simulink model "sim_att_dist_obs_tie_2020"  (R2020a)
settings: Solver=ode4  StartTime=0.0  StopTime=30.0  FixedStep=0.01  RelTol=1e-3
values from neighbouring files (symbols this model uses):
  beta_Phi_1 = pp0 * cal_frac_squ( 3, p_p0_plus_1, q_p0_plus_1 )                          * cal_frac_squ( eps_s_bar / pi, p_p0_min_2, q_p0_min_2 )                          / ( 2 * ( 2 * pp0 - 1 ) * tanh( gamma0 * ( eps_s_bar / pi ) / 2 ) )                          - ( cal_frac_squ( 3, p_p0_plus_1, q_p0_plus_1 ) * gamma0 / ( 4 * ( 2 * pp0 -1 ) ) )                          * cal_frac_squ( eps_s_bar / pi, p_p0_min_ ...(+136 chars)    [init_att_dist_obs_tie_2020.m]
  beta_Phi_2 = ( 1 - pp0 ) * cal_frac_squ( 3, p_p0_plus_1, q_p0_plus_1 )                          / ( 2 * ( 1 - 2 * pp0 ) * cal_frac_squ( eps_s_bar / pi, p_p0_0, q_p0_0 ) * tanh( gamma0 * ( eps_s_bar / pi ) / 2 ) )                          - ( cal_frac_squ( 3, p_p0_plus_1, q_p0_plus_1 ) * gamma0 / ( 4 * ( 1 - 2 * pp0 ) ) )                          * cal_frac_squ( eps_s_bar / pi, p_1_min_p0, q_1_min_p0 )          ...(+112 chars)    [init_att_dist_obs_tie_2020.m]
  c1_diff_ui = diag([25; 30; 20])    [init_att_dist_obs_tie_2020.m]
  c2_diff_ui = diag([50; 50; 10])    [init_att_dist_obs_tie_2020.m]
  c3_diff_ui = diag([15; 15; 10])    [init_att_dist_obs_tie_2020.m]
  c_w_1 = diag( [20; 15; 15] )    [init_att_dist_obs_tie_2020.m]
  c_w_2 = diag( [20; 15; 15] )    [init_att_dist_obs_tie_2020.m]
  c_w_3 = diag( [2; 2; 2] )    [init_att_dist_obs_tie_2020.m]
  cS0 = diag( [4.5; 4.5; 4.5] )    [init_att_dist_obs_tie_2020.m]
  dw_aa_t = 0.2 * ones(3, 5) + ( 1.0 - 0.2 ) * rand(3, 5)    [init_att_dist_obs_tie_2020.m]
  dw_ff_t = [ 0.4 * ones(1, 5) + ( 1.0 - 0.4 ) * rand(1, 5);                      0.4 * ones(1, 5) + ( 1.0 - 0.4 ) * rand(1, 5);                      0.2 * ones(1, 5) + ( 0.6 - 0.2 ) * rand(1, 5) ]    [init_att_dist_obs_tie_2020.m]
  dw_phi_t = ( - pi / 2 ) * ones(3, 5) + ( pi / 2 - ( - pi / 2 ) ) * rand(3, 5)    [init_att_dist_obs_tie_2020.m]
  dwci_init = zeros(3,5)    [init_att_dist_obs_tie_2020.m]
  eps_s_bar_div_pi = eps_s_bar / pi    (= 0.03)    [init_att_dist_obs_tie_2020.m]
  epw = [1; 1; 1]    [init_att_dist_obs_tie_2020.m]
  gamma0 = 20    [init_att_dist_obs_tie_2020.m]
  Ji = zeros(3,3,NF)    [init_att_dist_obs_tie_2020.m]
  k_J_0 = diag( [1; 1; 1] )    [init_att_dist_obs_tie_2020.m]
  kaiw = [10; 10; 10]    [init_att_dist_obs_tie_2020.m]
  l1w = [50; 50; 50]    [init_att_dist_obs_tie_2020.m]
  l2w = [60; 60; 60]    [init_att_dist_obs_tie_2020.m]
  Lamd_diff_ui = 0.8    [init_att_dist_obs_tie_2020.m]
  mu_c_theta = 100    [init_att_dist_obs_tie_2020.m]
  pos0 = zeros(3, 1)    [init_att_dist_obs_tie_2020.m]
  pp0 = 8 / 11    (= 0.727272727273)    [init_att_dist_obs_tie_2020.m]
  PZ0 = P0(3)    [init_att_dist_obs_tie_2020.m]
  PZ1 = 10    [init_att_dist_obs_tie_2020.m]
  Qci_init = repmat([1;0;0;0],1,NF)    [init_att_dist_obs_tie_2020.m]
  R0 = 4    [init_att_dist_obs_tie_2020.m]
  R1 = 8    [init_att_dist_obs_tie_2020.m]
  Rci_init = zeros(3,3,NF)    [init_att_dist_obs_tie_2020.m]
  Ri_init = zeros(3,3,NF)    [init_att_dist_obs_tie_2020.m]
  Rx2 = 10    [init_att_dist_obs_tie_2020.m]
  Ry2 = 6    [init_att_dist_obs_tie_2020.m]
  Rz2 = 4    [init_att_dist_obs_tie_2020.m]
  T0 = 0    [init_att_dist_obs_tie_2020.m]
  T1 = tseq1    (= 10)    [init_att_dist_obs_tie_2020.m]
  T2 = tseq1 + tseq12 + tseq2    (= 30)    [init_att_dist_obs_tie_2020.m]
  thr_p_plus_1 = cal_frac_squ( 3, p_p0_plus_1, q_p0_plus_1 )    [init_att_dist_obs_tie_2020.m]
  ui_init = zeros(3,NF)    [init_att_dist_obs_tie_2020.m]
  vel0 = zeros(3, 1)    [init_att_dist_obs_tie_2020.m]
  wci_init = zeros(3,5)    [init_att_dist_obs_tie_2020.m]
  zeta_diff_ui = 0.05    [init_att_dist_obs_tie_2020.m]
undefined symbols (not defined in the file or in its folder): cal_frac_squ, p_2_p0, p_beta_w_1, p_beta_w_2, p_p0_min_1, p_p0_plus_1, q_2_p0, q_beta_w_1, q_beta_w_2, q_p0_min_1, q_p0_plus_1, Qei_init, Qi_init, Rei_init, V_Phi_Rei_init, wei_init, wi_init
(part 3 of 4)

== matlab function sim_att_dist_obs_tie_2020/combine V_Phi_Rei_squ_2p ==
  data: V_Phi_Rei_squ_2p_node_1 input; V_Phi_Rei_squ_2p_node_2 input; V_Phi_Rei_squ_2p_node_3 input; V_Phi_Rei_squ_2p_node_4 input; V_Phi_Rei_squ_2p_node_5 input; V_Phi_Rei_squ_2p_vec output
function V_Phi_Rei_squ_2p_vec  = fcn(V_Phi_Rei_squ_2p_node_1, V_Phi_Rei_squ_2p_node_2, V_Phi_Rei_squ_2p_node_3, ...
                                                                        V_Phi_Rei_squ_2p_node_4, V_Phi_Rei_squ_2p_node_5)
%%%% 合并姿态误差指数坐标
V_Phi_Rei_squ_2p_vec = zeros(3,5);
V_Phi_Rei_squ_2p_vec(:,1) = V_Phi_Rei_squ_2p_node_1(:);
V_Phi_Rei_squ_2p_vec(:,2) = V_Phi_Rei_squ_2p_node_2(:);
V_Phi_Rei_squ_2p_vec(:,3) = V_Phi_Rei_squ_2p_node_3(:);
V_Phi_Rei_squ_2p_vec(:,4) = V_Phi_Rei_squ_2p_node_4(:);
V_Phi_Rei_squ_2p_vec(:,5) = V_Phi_Rei_squ_2p_node_5(:);

== matlab function sim_att_dist_obs_tie_2020/combine V_Phi_Rei_squ_p_min_1 ==
  data: V_Phi_Rei_squ_p_min_1_node_1 input; V_Phi_Rei_squ_p_min_1_node_2 input; V_Phi_Rei_squ_p_min_1_node_3 input; V_Phi_Rei_squ_p_min_1_node_4 input; V_Phi_Rei_squ_p_min_1_node_5 input; V_Phi_Rei_squ_p_min_1_vec output
function V_Phi_Rei_squ_p_min_1_vec  = fcn(V_Phi_Rei_squ_p_min_1_node_1, V_Phi_Rei_squ_p_min_1_node_2, V_Phi_Rei_squ_p_min_1_node_3, ...
                                                                                V_Phi_Rei_squ_p_min_1_node_4, V_Phi_Rei_squ_p_min_1_node_5)
%%%% 合并姿态误差导数
V_Phi_Rei_squ_p_min_1_vec = zeros(3,5);
V_Phi_Rei_squ_p_min_1_vec(:,1) = V_Phi_Rei_squ_p_min_1_node_1(:);
V_Phi_Rei_squ_p_min_1_vec(:,2) = V_Phi_Rei_squ_p_min_1_node_2(:);
V_Phi_Rei_squ_p_min_1_vec(:,3) = V_Phi_Rei_squ_p_min_1_node_3(:);
V_Phi_Rei_squ_p_min_1_vec(:,4) = V_Phi_Rei_squ_p_min_1_node_4(:);
V_Phi_Rei_squ_p_min_1_vec(:,5) = V_Phi_Rei_squ_p_min_1_node_5(:);

== matlab function sim_att_dist_obs_tie_2020/cal neso x1_hat agent 3 ==
  data: l1w input; epw input; Ji input; x1_hat_vec input; dw_hat_vec input; wi_vec input; d_x1_hat_3 output; taui_vec input
function d_x1_hat_3 = fcn(l1w, epw, Ji, x1_hat_vec, dw_hat_vec, wi_vec, taui_vec)
%%%% 计算扰动观测中间变量
iiuav = 3;
d_x1_hat_3 = dw_hat_vec(:,iiuav) + (l1w ./ epw) .* (Ji(:,:,iiuav) * wi_vec(:,iiuav) - x1_hat_vec(:,iiuav)) ...
                        + ( -cal_askew_mat(wi_vec(:,iiuav)) * Ji(:,:,iiuav) * wi_vec(:,iiuav) + taui_vec(:,iiuav) );

== matlab function sim_att_dist_obs_tie_2020/combine V_Phi_Rei_squ_p_plus_1 ==
  data: V_Phi_Rei_squ_p_plus_1_node_1 input; V_Phi_Rei_squ_p_plus_1_node_2 input; V_Phi_Rei_squ_p_plus_1_node_3 input; V_Phi_Rei_squ_p_plus_1_node_4 input; V_Phi_Rei_squ_p_plus_1_node_5 input; V_Phi_Rei_squ_p_plus_1_vec output
function V_Phi_Rei_squ_p_plus_1_vec  = fcn(V_Phi_Rei_squ_p_plus_1_node_1, V_Phi_Rei_squ_p_plus_1_node_2, V_Phi_Rei_squ_p_plus_1_node_3, ...
                                                                                V_Phi_Rei_squ_p_plus_1_node_4, V_Phi_Rei_squ_p_plus_1_node_5)
%%%% 合并姿态误差指数坐标
V_Phi_Rei_squ_p_plus_1_vec = zeros(3,5);
V_Phi_Rei_squ_p_plus_1_vec(:,1) = V_Phi_Rei_squ_p_plus_1_node_1(:);
V_Phi_Rei_squ_p_plus_1_vec(:,2) = V_Phi_Rei_squ_p_plus_1_node_2(:);
V_Phi_Rei_squ_p_plus_1_vec(:,3) = V_Phi_Rei_squ_p_plus_1_node_3(:);
V_Phi_Rei_squ_p_plus_1_vec(:,4) = V_Phi_Rei_squ_p_plus_1_node_4(:);
V_Phi_Rei_squ_p_plus_1_vec(:,5) = V_Phi_Rei_squ_p_plus_1_node_5(:);

== matlab function sim_att_dist_obs_tie_2020/combine duihat d2uihat ==
  data: d_ui_hat_node_1 input; duihat_vec output; d2uihat_vec output; d_ui_hat_node_2 input; d_ui_hat_node_3 input; d_ui_hat_node_4 input; d_ui_hat_node_5 input; d2_ui_hat_node_1 input; d2_ui_hat_node_2 input; d2_ui_hat_node_3 input; d2_ui_hat_node_4 input; d2_ui_hat_node_5 input
function [duihat_vec, d2uihat_vec] = fcn(d_ui_hat_node_1, d_ui_hat_node_2, d_ui_hat_node_3, d_ui_hat_node_4, d_ui_hat_node_5, ...
                                                                            d2_ui_hat_node_1, d2_ui_hat_node_2, d2_ui_hat_node_3, d2_ui_hat_node_4, d2_ui_hat_node_5)

duihat_vec = [d_ui_hat_node_1(:), d_ui_hat_node_2(:), d_ui_hat_node_3(:), d_ui_hat_node_4(:), d_ui_hat_node_5(:)];
d2uihat_vec = [d2_ui_hat_node_1(:), d2_ui_hat_node_2(:), d2_ui_hat_node_3(:), d2_ui_hat_node_4(:), d2_ui_hat_node_5(:)];

== matlab function sim_att_dist_obs_tie_2020/combine dwi ==
  data: wi_1 input; wi_vec output; wi_2 input; wi_3 input; wi_4 input; wi_5 input
function wi_vec = fcn(wi_1, wi_2, wi_3, wi_4, wi_5)
%%%% 合并姿态角速率
wi_vec = [wi_1(:), wi_2(:), wi_3(:), wi_4(:), wi_5(:)];

== matlab function sim_att_dist_obs_tie_2020/combine tau ==
  data: tau_1 input; taui_vec output; tau_2 input; tau_3 input; tau_4 input; tau_5 input
function taui_vec = fcn(tau_1, tau_2, tau_3, tau_4, tau_5)
%%%% 合并辅助姿态角速率
taui_vec = [tau_1(:), tau_2(:), tau_3(:), tau_4(:), tau_5(:)];

== matlab function sim_att_dist_obs_tie_2020/combine tau1 ==
  data: dw_1 input; dw_vec output; dw_2 input; dw_3 input; dw_4 input; dw_5 input
function dw_vec = fcn(dw_1, dw_2, dw_3, dw_4, dw_5)
%%%% 合并辅助姿态角速率
dw_vec = [dw_1(:), dw_2(:), dw_3(:), dw_4(:), dw_5(:)];

== matlab function sim_att_dist_obs_tie_2020/combine theta_Si_beta_w_1 ==
  data: theta_Si_beta_w_1_node_1 input; theta_Si_beta_w_1_node_2 input; theta_Si_beta_w_1_node_3 input; theta_Si_beta_w_1_node_4 input; theta_Si_beta_w_1_node_5 input; theta_Si_beta_w_1_vec output
function theta_Si_beta_w_1_vec  = fcn(theta_Si_beta_w_1_node_1, theta_Si_beta_w_1_node_2, theta_Si_beta_w_1_node_3, ...
                                                                        theta_Si_beta_w_1_node_4, theta_Si_beta_w_1_node_5)
%%%% 合并误差非线性项
theta_Si_beta_w_1_vec = zeros(3,5);
theta_Si_beta_w_1_vec(:,1) = theta_Si_beta_w_1_node_1(:);
theta_Si_beta_w_1_vec(:,2) = theta_Si_beta_w_1_node_2(:);
theta_Si_beta_w_1_vec(:,3) = theta_Si_beta_w_1_node_3(:);
theta_Si_beta_w_1_vec(:,4) = theta_Si_beta_w_1_node_4(:);
theta_Si_beta_w_1_vec(:,5) = theta_Si_beta_w_1_node_5(:);

== matlab function sim_att_dist_obs_tie_2020/combine theta_Si_beta_w_2 ==
  data: theta_Si_beta_w_2_node_1 input; theta_Si_beta_w_2_node_2 input; theta_Si_beta_w_2_node_3 input; theta_Si_beta_w_2_node_4 input; theta_Si_beta_w_2_node_5 input; theta_Si_beta_w_2_vec output
function theta_Si_beta_w_2_vec  = fcn(theta_Si_beta_w_2_node_1, theta_Si_beta_w_2_node_2, theta_Si_beta_w_2_node_3, ...
                                                                        theta_Si_beta_w_2_node_4, theta_Si_beta_w_2_node_5)
%%%% 合并误差非线性项
theta_Si_beta_w_2_vec = zeros(3,5);
theta_Si_beta_w_2_vec(:,1) = theta_Si_beta_w_2_node_1(:);
theta_Si_beta_w_2_vec(:,2) = theta_Si_beta_w_2_node_2(:);
theta_Si_beta_w_2_vec(:,3) = theta_Si_beta_w_2_node_3(:);
theta_Si_beta_w_2_vec(:,4) = theta_Si_beta_w_2_node_4(:);
theta_Si_beta_w_2_vec(:,5) = theta_Si_beta_w_2_node_5(:);

== matlab function sim_att_dist_obs_tie_2020/combine wci dwci ==
  data: wci_node_1 input; wci_vec output; wci_node_2 input; wci_node_3 input; wci_node_4 input; wci_node_5 input; dwci_vec output; dwci_node_1 input; dwci_node_2 input; dwci_node_3 input; dwci_node_4 input; dwci_node_5 input
function [wci_vec, dwci_vec] = fcn(wci_node_1, wci_node_2, wci_node_3, wci_node_4, wci_node_5, ...
                                                                dwci_node_1, dwci_node_2, dwci_node_3, dwci_node_4, dwci_node_5)
%%%% 合并姿态角速率指令及其导数
wci_vec = [wci_node_1(:), wci_node_2(:), wci_node_3(:), wci_node_4(:), wci_node_5(:)];
dwci_vec = [dwci_node_1(:), dwci_node_2(:), dwci_node_3(:), dwci_node_4(:), dwci_node_5(:)];

== matlab function sim_att_dist_obs_tie_2020/combine wei Qei Rei ==
  data: wei_1 input; wei_vec output; wei_2 input; wei_3 input; wei_4 input; wei_5 input; Qei_1 input; Qei_2 input; Qei_3 input; Qei_4 input; Qei_5 input; Rei_1 input; Rei_2 input; Rei_3 input; Rei_4 input; Rei_5 input; Qei_vec output; Rei_vec output
function [wei_vec, Qei_vec, Rei_vec] = fcn(wei_1, wei_2, wei_3, wei_4, wei_5, ...
                                                                            Qei_1, Qei_2, Qei_3, Qei_4, Qei_5, ...
                                                                            Rei_1, Rei_2, Rei_3, Rei_4, Rei_5)
%%%% 合并姿态角速率误差/四元数误差/姿态旋转矩阵误差
wei_vec = zeros(3,5);
wei_vec(:,1) = wei_1(:);
wei_vec(:,2) = wei_2(:);
wei_vec(:,3) = wei_3(:);
wei_vec(:,4) = wei_4(:);
wei_vec(:,5) = wei_5(:);

Qei_vec = zeros(4,5);
Qei_vec(:,1) = Qei_1(:);
Qei_vec(:,2) = Qei_2(:);
Qei_vec(:,3) = Qei_3(:);
Qei_vec(:,4) = Qei_4(:);
Qei_vec(:,5) = Qei_5(:);

Rei_vec = zeros(3,3,5);
Rei_vec(:,:,1) = Rei_1;
Rei_vec(:,:,2) = Rei_2;
Rei_vec(:,:,3) = Rei_3;
Rei_vec(:,:,4) = Rei_4;
Rei_vec(:,:,5) = Rei_5;

== matlab function sim_att_dist_obs_tie_2020/cal neso x1_hat agent 4 ==
  data: l1w input; epw input; Ji input; x1_hat_vec input; dw_hat_vec input; wi_vec input; d_x1_hat_4 output; taui_vec input
function d_x1_hat_4 = fcn(l1w, epw, Ji, x1_hat_vec, dw_hat_vec, wi_vec, taui_vec)
%%%% 计算扰动观测中间变量
iiuav = 4;
d_x1_hat_4 = dw_hat_vec(:,iiuav) + (l1w ./ epw) .* (Ji(:,:,iiuav) * wi_vec(:,iiuav) - x1_hat_vec(:,iiuav)) ...
                        + ( -cal_askew_mat(wi_vec(:,iiuav)) * Ji(:,:,iiuav) * wi_vec(:,iiuav) + taui_vec(:,iiuav) );

== matlab function sim_att_dist_obs_tie_2020/generate angular rate disturbance agent 1 ==
  data: dw_1 output; dw_aa_t input; dw_ff_t input; dw_phi_t input; t input
function dw_1 = fcn(dw_aa_t, dw_ff_t, dw_phi_t, t)
%%%% 姿态动力学方程中的扰动项设置
epsil_t = zeros(3, 1);

for kk = 1:5
    epsil_t = epsil_t + dw_aa_t(:, kk) .* sin( 2 * pi * dw_ff_t(:, kk) * t + dw_phi_t(:, kk) );
end

dw_1 = [ epsil_t(1) + 1.6 * sin( 0.4 * t ) + 2.0 * cos( 0.5 * t ) + 1.4 * sin( 0.7 * t ) ...
                + 4 * exp( -0.1 * t ) * sin( 0.8 * t ) + 3 / ( 1 + exp( -0.2 * ( t - 15 ) ) ); ...
                epsil_t(2) + 1.2 * sin( 0.2 * t ) + 3 * cos( 0.4 * t ) + 0.8 * sin( 0.6 * t ) ...
                + 2 * exp( -0.15 * t ) * cos( 1.2 * t ) + 3 / ( 1 + exp( -0.3 * ( t - 25 ) ) ); ...
                epsil_t(3) + 1.8 * sin( 0.2 * t ) + 1.6 * sin( 0.3 * t ) + 1.6 * cos( 0.4 * t ) ...
                + 4 * exp( -0.05 * t ) * sin( 0.5 * t + pi / 4 ) + 3 / ( 1 + exp( -0.5 * ( t - 20 ) ) ) ];

== matlab function sim_att_dist_obs_tie_2020/generate angular rate disturbance agent 2 ==
  data: dw_2 output; dw_aa_t input; dw_ff_t input; dw_phi_t input; t input
function dw_2 = fcn(dw_aa_t, dw_ff_t, dw_phi_t, t)
%%%% 姿态动力学方程中的扰动项设置
epsil_t = zeros(3, 1);

for kk = 1:5
    epsil_t = epsil_t + dw_aa_t(:, kk) .* sin( 2 * pi * dw_ff_t(:, kk) * t + dw_phi_t(:, kk) );
end

dw_2 = [ epsil_t(1) + 1.6 * sin( 0.2 * t ) + 2.0 * cos( 0.3 * t ) + 1.4 * sin( 0.5 * t ) ...
                + 4 * exp( -0.1 * t ) * sin( 0.5 * t ) + 3 / ( 1 + exp( -0.2 * ( t - 15 ) ) ); ...
                epsil_t(2) + 1.2 * sin( 0.1 * t ) + 3 * cos( 0.2 * t ) + 0.8 * sin( 0.4 * t ) ...
                + 2 * exp( -0.15 * t ) * cos( 0.6 * t ) + 3 / ( 1 + exp( -0.3 * ( t - 25 ) ) ); ...
                epsil_t(3) + 1.8 * sin( 0.1 * t ) + 1.6 * sin( 0.2 * t ) + 1.6 * cos( 0.3 * t ) ...
                + 4 * exp( -0.05 * t ) * sin( 0.4 * t + pi / 4 ) + 3 / ( 1 + exp( -0.5 * ( t - 20 ) ) ) ];

== matlab function sim_att_dist_obs_tie_2020/generate angular rate disturbance agent 3 ==
  data: dw_3 output; dw_aa_t input; dw_ff_t input; dw_phi_t input; t input
function dw_3 = fcn(dw_aa_t, dw_ff_t, dw_phi_t, t)
%%%% 姿态动力学方程中的扰动项设置
epsil_t = zeros(3, 1);

for kk = 1:5
    epsil_t = epsil_t + dw_aa_t(:, kk) .* sin( 2 * pi * dw_ff_t(:, kk) * t + dw_phi_t(:, kk) );
end

dw_3 = [ epsil_t(1) + 1.6 * sin( 0.2 * t ) + 2.0 * cos( 0.3 * t ) + 1.4 * sin( 0.5 * t ) ...
                + 4 * exp( -0.1 * t ) * sin( 0.5 * t ) + 3 / ( 1 + exp( -0.2 * ( t - 15 ) ) ); ...
                epsil_t(2) + 1.2 * sin( 0.1 * t ) + 3 * cos( 0.2 * t ) + 0.8 * sin( 0.4 * t ) ...
                + 2 * exp( -0.15 * t ) * cos( 0.6 * t ) + 3 / ( 1 + exp( -0.3 * ( t - 25 ) ) ); ...
                epsil_t(3) + 1.8 * sin( 0.1 * t ) + 1.6 * sin( 0.2 * t ) + 1.6 * cos( 0.3 * t ) ...
                + 4 * exp( -0.05 * t ) * sin( 0.4 * t + pi / 4 ) + 3 / ( 1 + exp( -0.5 * ( t - 20 ) ) ) ];

== matlab function sim_att_dist_obs_tie_2020/generate angular rate disturbance agent 4 ==
  data: dw_4 output; dw_aa_t input; dw_ff_t input; dw_phi_t input; t input
function dw_4 = fcn(dw_aa_t, dw_ff_t, dw_phi_t, t)
%%%% 姿态动力学方程中的扰动项设置
epsil_t = zeros(3, 1);

for kk = 1:5
    epsil_t = epsil_t + dw_aa_t(:, kk) .* sin( 2 * pi * dw_ff_t(:, kk) * t + dw_phi_t(:, kk) );
end

dw_4 = [ epsil_t(1) + 1.6 * sin( 0.2 * t ) + 2.0 * cos( 0.3 * t ) + 1.4 * sin( 0.5 * t ) ...
                + 4 * exp( -0.1 * t ) * sin( 0.5 * t ) + 3 / ( 1 + exp( -0.2 * ( t - 15 ) ) ); ...
                epsil_t(2) + 1.2 * sin( 0.1 * t ) + 3 * cos( 0.2 * t ) + 0.8 * sin( 0.4 * t ) ...
                + 2 * exp( -0.15 * t ) * cos( 0.6 * t ) + 3 / ( 1 + exp( -0.3 * ( t - 25 ) ) ); ...
                epsil_t(3) + 1.8 * sin( 0.1 * t ) + 1.6 * sin( 0.2 * t ) + 1.6 * cos( 0.3 * t ) ...
                + 4 * exp( -0.05 * t ) * sin( 0.4 * t + pi / 4 ) + 3 / ( 1 + exp( -0.5 * ( t - 20 ) ) ) ];

== matlab function sim_att_dist_obs_tie_2020/generate angular rate disturbance agent 5 ==
  data: dw_5 output; dw_aa_t input; dw_ff_t input; dw_phi_t input; t input
function dw_5 = fcn(dw_aa_t, dw_ff_t, dw_phi_t, t)
%%%% 姿态动力学方程中的扰动项设置
epsil_t = zeros(3, 1);

for kk = 1:5
    epsil_t = epsil_t + dw_aa_t(:, kk) .* sin( 2 * pi * dw_ff_t(:, kk) * t + dw_phi_t(:, kk) );
end

dw_5 = [ epsil_t(1) + 1.6 * sin( 0.2 * t ) + 2.0 * cos( 0.3 * t ) + 1.4 * sin( 0.5 * t ) ...
                + 4 * exp( -0.1 * t ) * sin( 0.5 * t ) + 3 / ( 1 + exp( -0.2 * ( t - 15 ) ) ); ...
                epsil_t(2) + 1.2 * sin( 0.1 * t ) + 3 * cos( 0.2 * t ) + 0.8 * sin( 0.4 * t ) ...
                + 2 * exp( -0.15 * t ) * cos( 0.6 * t ) + 3 / ( 1 + exp( -0.3 * ( t - 25 ) ) ); ...
                epsil_t(3) + 1.8 * sin( 0.1 * t ) + 1.6 * sin( 0.2 * t ) + 1.6 * cos( 0.3 * t ) ...
                + 4 * exp( -0.05 * t ) * sin( 0.4 * t + pi / 4 ) + 3 / ( 1 + exp( -0.5 * ( t - 20 ) ) ) ];

== matlab function sim_att_dist_obs_tie_2020/trans to column100 ==
  data: x input; y output
function y = fcn(x)
y = x(:);

== matlab function sim_att_dist_obs_tie_2020/trans to column101 ==
  data: x input; y output
function y = fcn(x)
y = x(:);

== matlab function sim_att_dist_obs_tie_2020/trans to column102 ==
  data: x input; y output
function y = fcn(x)
y = x(:);

== matlab function sim_att_dist_obs_tie_2020/trans to column103 ==
  data: x input; y output
function y = fcn(x)
y = x(:);

== matlab function sim_att_dist_obs_tie_2020/trans to column104 ==
  data: x input; y output
function y = fcn(x)
y = x(:);

== matlab function sim_att_dist_obs_tie_2020/trans to column105 ==
  data: x input; y output
function y = fcn(x)
y = x(:);

== matlab function sim_att_dist_obs_tie_2020/trans to column106 ==
  data: x input; y output
function y = fcn(x)
y = x(:);

== matlab function sim_att_dist_obs_tie_2020/trans to column116 ==
  data: x input; y output
function y = fcn(x)
y = x(:);

== matlab function sim_att_dist_obs_tie_2020/trans to column118 ==
  data: x input; y output
function y = fcn(x)
y = x(:);

== matlab function sim_att_dist_obs_tie_2020/trans to column119 ==
  data: x input; y output
function y = fcn(x)
y = x(:);

== matlab function sim_att_dist_obs_tie_2020/trans to column120 ==
  data: x input; y output
function y = fcn(x)
y = x(:);

== matlab function sim_att_dist_obs_tie_2020/trans to column121 ==
  data: x input; y output
function y = fcn(x)
y = x(:);

== matlab function sim_att_dist_obs_tie_2020/cal neso x1_hat agent 5 ==
  data: l1w input; epw input; Ji input; x1_hat_vec input; dw_hat_vec input; wi_vec input; d_x1_hat_5 output; taui_vec input
function d_x1_hat_5 = fcn(l1w, epw, Ji, x1_hat_vec, dw_hat_vec, wi_vec, taui_vec)
%%%% 计算扰动观测中间变量
iiuav = 5;
d_x1_hat_5 = dw_hat_vec(:,iiuav) + (l1w ./ epw) .* (Ji(:,:,iiuav) * wi_vec(:,iiuav) - x1_hat_vec(:,iiuav)) ...
                        + ( -cal_askew_mat(wi_vec(:,iiuav)) * Ji(:,:,iiuav) * wi_vec(:,iiuav) + taui_vec(:,iiuav) );

== matlab function sim_att_dist_obs_tie_2020/trans to column122 ==
  data: x input; y output
function y = fcn(x)
y = x(:);

== matlab function sim_att_dist_obs_tie_2020/trans to column123 ==
  data: x input; y output
function y = fcn(x)
y = x(:);

== matlab function sim_att_dist_obs_tie_2020/trans to column124 ==
  data: x input; y output
function y = fcn(x)
y = x(:);

== matlab function sim_att_dist_obs_tie_2020/trans to column125 ==
  data: x input; y output
function y = fcn(x)
y = x(:);

== matlab function sim_att_dist_obs_tie_2020/trans to column61 ==
  data: x input; y output
function y = fcn(x)
y = x(:);

== matlab function sim_att_dist_obs_tie_2020/trans to column62 ==
  data: x input; y output
function y = fcn(x)
y = x(:);

== matlab function sim_att_dist_obs_tie_2020/trans to column63 ==
  data: x input; y output
function y = fcn(x)
y = x(:);

== matlab function sim_att_dist_obs_tie_2020/trans to column64 ==
  data: x input; y output
function y = fcn(x)
y = x(:);

== matlab function sim_att_dist_obs_tie_2020/trans to column65 ==
  data: x input; y output
function y = fcn(x)
y = x(:);

== matlab function sim_att_dist_obs_tie_2020/trans to column66 ==
  data: x input; y output
function y = fcn(x)
y = x(:);

== matlab function sim_att_dist_obs_tie_2020/trans to column67 ==
  data: x input; y output
function y = fcn(x)
y = x(:);

== matlab function sim_att_dist_obs_tie_2020/trans to column68 ==
  data: x input; y output
function y = fcn(x)
y = x(:);

== matlab function sim_att_dist_obs_tie_2020/trans to column69 ==
  data: x input; y output
function y = fcn(x)
y = x(:);

== matlab function sim_att_dist_obs_tie_2020/trans to column70 ==
  data: x input; y output
function y = fcn(x)
y = x(:);

== matlab function sim_att_dist_obs_tie_2020/trans to column71 ==
  data: x input; y output
function y = fcn(x)
y = x(:);

== matlab function sim_att_dist_obs_tie_2020/trans to column72 ==
  data: x input; y output
function y = fcn(x)
y = x(:);

== matlab function sim_att_dist_obs_tie_2020/trans to column73 ==
  data: x input; y output
function y = fcn(x)
y = x(:);

== matlab function sim_att_dist_obs_tie_2020/trans to column74 ==
  data: x input; y output
function y = fcn(x)
y = x(:);

== matlab function sim_att_dist_obs_tie_2020/cal neso dw_hat agent 3 ==
  data: Ji input; l2w input; epw input; kaiw input; x1_hat_vec input; wi_vec input; d_dw_hat_3 output
function d_dw_hat_3 = fcn(Ji, l2w, epw, kaiw, x1_hat_vec, wi_vec)
%%%% 计算扰动观测值
iiuav = 3;
del_x1 = (kaiw ./ epw) .* ( Ji(:,:,iiuav) * wi_vec(:,iiuav) - x1_hat_vec(:,iiuav) );
phi_del_x1 = zeros(3,1);
for jj = 1:length(del_x1)
    if del_x1(jj,1) <= -pi/2
        phi_del_x1(jj,1) = -1;
    elseif del_x1(jj,1) >= pi/2
        phi_del_x1(jj,1) = 1;
    else
        phi_del_x1(jj,1) = sin(del_x1(jj,1));
    end
end
d_dw_hat_3 = (l2w ./ (epw.^2)) .* (Ji(:,:,iiuav) * wi_vec(:,iiuav) - x1_hat_vec(:,iiuav)) ...
                            + (1 ./ epw) .* phi_del_x1;

== matlab function sim_att_dist_obs_tie_2020/trans to column75 ==
  data: x input; y output
function y = fcn(x)
y = x(:);

== matlab function sim_att_dist_obs_tie_2020/trans to column76 ==
  data: x input; y output
function y = fcn(x)
y = x(:);

== matlab function sim_att_dist_obs_tie_2020/trans to column77 ==
  data: x input; y output
function y = fcn(x)
y = x(:);

== matlab function sim_att_dist_obs_tie_2020/trans to column78 ==
  data: x input; y output
function y = fcn(x)
y = x(:);

== matlab function sim_att_dist_obs_tie_2020/trans to column79 ==
  data: x input; y output
function y = fcn(x)
y = x(:);

== matlab function sim_att_dist_obs_tie_2020/trans to column80 ==
  data: x input; y output
function y = fcn(x)
y = x(:);

== matlab function sim_att_dist_obs_tie_2020/trans to column81 ==
  data: x input; y output
function y = fcn(x)
y = x(:);

== matlab function sim_att_dist_obs_tie_2020/trans to column82 ==
  data: x input; y output
function y = fcn(x)
y = x(:);

== matlab function sim_att_dist_obs_tie_2020/trans to column83 ==
  data: x input; y output
function y = fcn(x)
y = x(:);

== matlab function sim_att_dist_obs_tie_2020/trans to column84 ==
  data: x input; y output
function y = fcn(x)
y = x(:);

== matlab function sim_att_dist_obs_tie_2020/trans to column85 ==
  data: x input; y output
function y = fcn(x)
y = x(:);

== matlab function sim_att_dist_obs_tie_2020/trans to column86 ==
  data: x input; y output
function y = fcn(x)
y = x(:);

== matlab function sim_att_dist_obs_tie_2020/trans to column87 ==
  data: x input; y output
function y = fcn(x)
y = x(:);

== matlab function sim_att_dist_obs_tie_2020/trans to column88 ==
  data: x input; y output
function y = fcn(x)
y = x(:);

== matlab function sim_att_dist_obs_tie_2020/trans to column89 ==
  data: x input; y output
function y = fcn(x)
y = x(:);

== matlab function sim_att_dist_obs_tie_2020/trans to column90 ==
  data: x input; y output
function y = fcn(x)
y = x(:);

== matlab function sim_att_dist_obs_tie_2020/trans to column91 ==
  data: x input; y output
function y = fcn(x)
y = x(:);

== matlab function sim_att_dist_obs_tie_2020/cal neso dw_hat agent 4 ==
  data: Ji input; l2w input; epw input; kaiw input; x1_hat_vec input; wi_vec input; d_dw_hat_4 output
function d_dw_hat_4 = fcn(Ji, l2w, epw, kaiw, x1_hat_vec, wi_vec)
%%%% 计算扰动观测值
iiuav = 4;
del_x1 = (kaiw ./ epw) .* ( Ji(:,:,iiuav) * wi_vec(:,iiuav) - x1_hat_vec(:,iiuav) );
phi_del_x1 = zeros(3,1);
for jj = 1:length(del_x1)
    if del_x1(jj,1) <= -pi/2
        phi_del_x1(jj,1) = -1;
    elseif del_x1(jj,1) >= pi/2
        phi_del_x1(jj,1) = 1;
    else
        phi_del_x1(jj,1) = sin(del_x1(jj,1));
    end
end
d_dw_hat_4 = (l2w ./ (epw.^2)) .* (Ji(:,:,iiuav) * wi_vec(:,iiuav) - x1_hat_vec(:,iiuav)) ...
                            + (1 ./ epw) .* phi_del_x1;

== matlab function sim_att_dist_obs_tie_2020/trans to column92 ==
  data: x input; y output
function y = fcn(x)
y = x(:);

== matlab function sim_att_dist_obs_tie_2020/trans to column93 ==
  data: x input; y output
function y = fcn(x)
y = x(:);

== matlab function sim_att_dist_obs_tie_2020/trans to column94 ==
  data: x input; y output
function y = fcn(x)
y = x(:);

== matlab function sim_att_dist_obs_tie_2020/trans to column95 ==
  data: x input; y output
function y = fcn(x)
y = x(:);

== matlab function sim_att_dist_obs_tie_2020/trans to column96 ==
  data: x input; y output
function y = fcn(x)
y = x(:);

== matlab function sim_att_dist_obs_tie_2020/trans to column97 ==
  data: x input; y output
function y = fcn(x)
y = x(:);

== matlab function sim_att_dist_obs_tie_2020/trans to column98 ==
  data: x input; y output
function y = fcn(x)
y = x(:);

== matlab function sim_att_dist_obs_tie_2020/trans to column99 ==
  data: x input; y output
function y = fcn(x)
y = x(:);

== matlab function sim_att_dist_obs_tie_2020/wi dynam agent 1 ==
  data: Ji input; dwi_1 output; wi_vec input; taui_vec input; dw_vec input
function dwi_1 = fcn(Ji, wi_vec, taui_vec, dw_vec)
%%%% 更新姿态角速率微分方程
iiuav = 1;
dwi_1 = inv(Ji(:,:,iiuav)) * ( -cal_askew_mat(wi_vec(:,iiuav)) * Ji(:,:,iiuav) * wi_vec(:,iiuav) ... 
                                                + taui_vec(:,iiuav) + dw_vec(:,iiuav) );

end

== matlab function sim_att_dist_obs_tie_2020/wi dynam agent 2 ==
  data: Ji input; dwi_2 output; wi_vec input; taui_vec input; dw_vec input
function dwi_2 = fcn(Ji, wi_vec, taui_vec, dw_vec)
%%%% 更新姿态角速率微分方程
iiuav = 2;
dwi_2 = inv(Ji(:,:,iiuav)) * ( -cal_askew_mat(wi_vec(:,iiuav)) * Ji(:,:,iiuav) * wi_vec(:,iiuav) ... 
                                                + taui_vec(:,iiuav) + dw_vec(:,iiuav) );

end

== matlab function sim_att_dist_obs_tie_2020/wi dynam agent 3 ==
  data: Ji input; dwi_3 output; wi_vec input; taui_vec input; dw_vec input
function dwi_3 = fcn(Ji, wi_vec, taui_vec, dw_vec)
%%%% 更新姿态角速率微分方程
iiuav = 3;
dwi_3 = inv(Ji(:,:,iiuav)) * ( -cal_askew_mat(wi_vec(:,iiuav)) * Ji(:,:,iiuav) * wi_vec(:,iiuav) ...
                                                + taui_vec(:,iiuav) + dw_vec(:,iiuav) );

end

== matlab function sim_att_dist_obs_tie_2020/wi dynam agent 4 ==
  data: Ji input; dwi_4 output; wi_vec input; taui_vec input; dw_vec input
function dwi_4 = fcn(Ji, wi_vec, taui_vec, dw_vec)
%%%% 更新姿态角速率微分方程
iiuav = 4;
dwi_4 = inv(Ji(:,:,iiuav)) * ( -cal_askew_mat(wi_vec(:,iiuav)) * Ji(:,:,iiuav) * wi_vec(:,iiuav) ...
                                                + taui_vec(:,iiuav) + dw_vec(:,iiuav) );

end

== matlab function sim_att_dist_obs_tie_2020/wi dynam agent 5 ==
  data: Ji input; dwi_5 output; wi_vec input; taui_vec input; dw_vec input
function dwi_5 = fcn(Ji, wi_vec, taui_vec, dw_vec)
%%%% 更新姿态角速率微分方程
iiuav = 5;
dwi_5 = inv(Ji(:,:,iiuav)) * ( -cal_askew_mat(wi_vec(:,iiuav)) * Ji(:,:,iiuav) * wi_vec(:,iiuav) ...
                                                + taui_vec(:,iiuav) + dw_vec(:,iiuav) );

end

== matlab function sim_att_dist_obs_tie_2020/combine norminal formation control input ==
  data: ui_1 input; ui_vec output; ui_2 input; ui_3 input; ui_4 input; ui_5 input
function ui_vec = fcn(ui_1, ui_2, ui_3, ui_4, ui_5)
%%%% 合并领导者编队跟踪误差结果
ui_vec = [ui_1(:), ui_2(:), ui_3(:), ui_4(:), ui_5(:)];

== matlab function sim_att_dist_obs_tie_2020/control input generator agent 1 ==
  data: u0 input; ui output
function ui  = fcn(u0)
%%%% 给出领导者参考加速度控制输入
g0 = 9.80663;
e3 = [0;0;1];

ui = g0 * e3 + u0(:);

== matlab function sim_att_dist_obs_tie_2020/cal neso dw_hat agent 5 ==
  data: Ji input; l2w input; epw input; kaiw input; x1_hat_vec input; wi_vec input; d_dw_hat_5 output
function d_dw_hat_5 = fcn(Ji, l2w, epw, kaiw, x1_hat_vec, wi_vec)
%%%% 计算扰动观测值
iiuav = 5;
del_x1 = (kaiw ./ epw) .* ( Ji(:,:,iiuav) * wi_vec(:,iiuav) - x1_hat_vec(:,iiuav) );
phi_del_x1 = zeros(3,1);
for jj = 1:length(del_x1)
    if del_x1(jj,1) <= -pi/2
        phi_del_x1(jj,1) = -1;
    elseif del_x1(jj,1) >= pi/2
        phi_del_x1(jj,1) = 1;
    else
        phi_del_x1(jj,1) = sin(del_x1(jj,1));
    end
end
d_dw_hat_5 = (l2w ./ (epw .^ 2)) .* (Ji(:,:,iiuav) * wi_vec(:,iiuav) - x1_hat_vec(:,iiuav)) ...
                            + (1 ./ epw) .* phi_del_x1;

== matlab function sim_att_dist_obs_tie_2020/control input generator agent 2 ==
  data: u0 input; ui output
function ui  = fcn(u0)
%%%% 给出领导者参考加速度控制输入
g0 = 9.80663;
e3 = [0;0;1];

ui = g0 * e3 + u0(:);

== matlab function sim_att_dist_obs_tie_2020/control input generator agent 3 ==
  data: u0 input; ui output
function ui  = fcn(u0)
%%%% 给出领导者参考加速度控制输入
g0 = 9.80663;
e3 = [0;0;1];

ui = g0 * e3 + u0(:);

== matlab function sim_att_dist_obs_tie_2020/control input generator agent 4 ==
  data: u0 input; ui output
function ui  = fcn(u0)
%%%% 给出领导者参考加速度控制输入
g0 = 9.80663;
e3 = [0;0;1];

ui = g0 * e3 + u0(:);

== matlab function sim_att_dist_obs_tie_2020/control input generator agent 5 ==
  data: u0 input; ui output
function ui  = fcn(u0)
%%%% 给出领导者参考加速度控制输入
g0 = 9.80663;
e3 = [0;0;1];

ui = g0 * e3 + u0(:);

== matlab function sim_att_dist_obs_tie_2020/cal error dw_tilt ==
  data: dw_vec input; dw_hat_vec input; dw_tilt_vec output
function dw_tilt_vec = fcn(dw_vec, dw_hat_vec)
%%%% 计算扰动观测误差dw_tilt
dw_tilt_vec = zeros(3,5);
for iiuav = 1:5
    dw_tilt_vec(:,iiuav) = dw_vec(:,iiuav) - dw_hat_vec(:,iiuav);
end

== matlab function sim_att_dist_obs_tie_2020/combine dw_hat ==
  data: dw_hat_1 input; dw_hat_2 input; dw_hat_3 input; dw_hat_4 input; dw_hat_5 input; dw_hat_vec output
function dw_hat_vec  = fcn(dw_hat_1, dw_hat_2, dw_hat_3, dw_hat_4, dw_hat_5)
%%%% 合并扰动观测值dw_hat
dw_hat_vec = [dw_hat_1(:), dw_hat_2(:), dw_hat_3(:), dw_hat_4(:), dw_hat_5(:)];

== matlab function sim_att_dist_obs_tie_2020/Qei dynam agent 3 ==
  data: Qei_vec input; dQei_3 output; wei_vec input
function dQei_3 = fcn(Qei_vec, wei_vec)
%%%% 更新四元数误差微分方程
iiuav = 3;

wei = wei_vec(:,iiuav);
thetaei = Qei_vec(1,iiuav);
qei = Qei_vec(2:4,iiuav);

GammaQei = zeros(4,3);
GammaQei(1,:) = -(qei');
GammaQei(2:4,:) = thetaei*eye(3,3) + cal_askew_mat(qei);
dQei_3 = (1/2)*GammaQei*wei;

end

== matlab function sim_att_dist_obs_tie_2020/Qei dynam agent 4 ==
  data: Qei_vec input; dQei_4 output; wei_vec input
function dQei_4 = fcn(Qei_vec, wei_vec)
%%%% 更新四元数误差微分方程
iiuav = 4;

wei = wei_vec(:,iiuav);
thetaei = Qei_vec(1,iiuav);
qei = Qei_vec(2:4,iiuav);

GammaQei = zeros(4,3);
GammaQei(1,:) = -(qei');
GammaQei(2:4,:) = thetaei*eye(3,3) + cal_askew_mat(qei);
dQei_4 = (1/2)*GammaQei*wei;

end

== matlab function sim_att_dist_obs_tie_2020/Qei dynam agent 5 ==
  data: Qei_vec input; dQei_5 output; wei_vec input
function dQei_5 = fcn(Qei_vec, wei_vec)
%%%% 更新四元数误差微分方程
iiuav = 5;

wei = wei_vec(:,iiuav);
thetaei = Qei_vec(1,iiuav);
qei = Qei_vec(2:4,iiuav);

GammaQei = zeros(4,3);
GammaQei(1,:) = -(qei');
GammaQei(2:4,:) = thetaei*eye(3,3) + cal_askew_mat(qei);
dQei_5 = (1/2)*GammaQei*wei;

end

== matlab function sim_att_dist_obs_tie_2020/Qi dynam agent 1 ==
  data: Qi_vec input; dQi_1 output; wi_vec input
function dQi_1 = fcn(Qi_vec, wi_vec)
%%%% 更新四元数微分方程
iiuav = 1;

wi = wi_vec(:,iiuav);
thetai = Qi_vec(1,iiuav);
qi = Qi_vec(2:4,iiuav);

GammaQi = zeros(4,3);
GammaQi(1,:) = -(qi');
GammaQi(2:4,:) = thetai*eye(3,3) + cal_askew_mat(qi);
dQi_1 = (1/2)*GammaQi*wi;

end

== matlab function sim_att_dist_obs_tie_2020/Qi dynam agent 2 ==
  data: Qi_vec input; dQi_2 output; wi_vec input
function dQi_2 = fcn(Qi_vec, wi_vec)
%%%% 更新四元数微分方程
iiuav = 2;

wi = wi_vec(:,iiuav);
thetai = Qi_vec(1,iiuav);
qi = Qi_vec(2:4,iiuav);

GammaQi = zeros(4,3);
GammaQi(1,:) = -(qi');
GammaQi(2:4,:) = thetai*eye(3,3) + cal_askew_mat(qi);
dQi_2 = (1/2)*GammaQi*wi;

end

== matlab function sim_att_dist_obs_tie_2020/Qi dynam agent 3 ==
  data: Qi_vec input; dQi_3 output; wi_vec input
function dQi_3 = fcn(Qi_vec, wi_vec)
%%%% 更新四元数微分方程
iiuav = 3;

wi = wi_vec(:,iiuav);
thetai = Qi_vec(1,iiuav);
qi = Qi_vec(2:4,iiuav);

GammaQi = zeros(4,3);
GammaQi(1,:) = -(qi');
GammaQi(2:4,:) = thetai*eye(3,3) + cal_askew_mat(qi);
dQi_3 = (1/2)*GammaQi*wi;

end

== matlab function sim_att_dist_obs_tie_2020/Qi dynam agent 4 ==
  data: Qi_vec input; dQi_4 output; wi_vec input
function dQi_4 = fcn(Qi_vec, wi_vec)
%%%% 更新四元数微分方程
iiuav = 4;

wi = wi_vec(:,iiuav);
thetai = Qi_vec(1,iiuav);
qi = Qi_vec(2:4,iiuav);

GammaQi = zeros(4,3);
GammaQi(1,:) = -(qi');
GammaQi(2:4,:) = thetai*eye(3,3) + cal_askew_mat(qi);
dQi_4 = (1/2)*GammaQi*wi;

end

== matlab function sim_att_dist_obs_tie_2020/Qi dynam agent 5 ==
  data: Qi_vec input; dQi_5 output; wi_vec input
function dQi_5 = fcn(Qi_vec, wi_vec)
%%%% 更新四元数微分方程
iiuav = 5;

wi = wi_vec(:,iiuav);
thetai = Qi_vec(1,iiuav);
qi = Qi_vec(2:4,iiuav);

GammaQi = zeros(4,3);
GammaQi(1,:) = -(qi');
GammaQi(2:4,:) = thetai*eye(3,3) + cal_askew_mat(qi);
dQi_5 = (1/2)*GammaQi*wi;

end

== matlab function sim_att_dist_obs_tie_2020/cal Fi_S agent 1 ==
  data: cS0 input; Ji input; wi_vec input; wci_vec input; wei_vec input; Fi_S_1 output; dwci_vec input; Rei_vec input; Phi_bar_psi_e_vec input
function Fi_S_1 = fcn(cS0, Ji, wi_vec, wci_vec, wei_vec, dwci_vec, Rei_vec, Phi_bar_psi_e_vec)
%%%% 计算补偿项
iiuav = 1;
Fi_S_1 = -cal_askew_mat( wi_vec(:,iiuav) ) * Ji(:,:,iiuav) * wi_vec(:,iiuav) ...
                + Ji(:,:,iiuav) * cal_askew_mat( wei_vec(:,iiuav) ) * ( Rei_vec(:,:,iiuav)' ) * wci_vec(:,iiuav) ...
                - Ji(:,:,iiuav) * ( Rei_vec(:,:,iiuav)' ) * dwci_vec(:,iiuav) ...
                + cS0 * Ji(:,:,iiuav) * Phi_bar_psi_e_vec(:,iiuav);

== matlab function sim_att_dist_obs_tie_2020/cal Fi_S agent 2 ==
  data: cS0 input; Ji input; wi_vec input; wci_vec input; wei_vec input; Fi_S_2 output; dwci_vec input; Rei_vec input; Phi_bar_psi_e_vec input
function Fi_S_2 = fcn(cS0, Ji, wi_vec, wci_vec, wei_vec, dwci_vec, Rei_vec, Phi_bar_psi_e_vec)
%%%% 计算补偿项
iiuav = 2;
Fi_S_2 = -cal_askew_mat( wi_vec(:,iiuav) ) * Ji(:,:,iiuav) * wi_vec(:,iiuav) ...
                + Ji(:,:,iiuav) * cal_askew_mat( wei_vec(:,iiuav) ) * ( Rei_vec(:,:,iiuav)' ) * wci_vec(:,iiuav) ...
                - Ji(:,:,iiuav) * ( Rei_vec(:,:,iiuav)' ) * dwci_vec(:,iiuav) ...
                + cS0 * Ji(:,:,iiuav) * Phi_bar_psi_e_vec(:,iiuav);

== matlab function sim_att_dist_obs_tie_2020/cal Fi_S agent 3 ==
  data: cS0 input; Ji input; wi_vec input; wci_vec input; wei_vec input; Fi_S_3 output; dwci_vec input; Rei_vec input; Phi_bar_psi_e_vec input
function Fi_S_3 = fcn(cS0, Ji, wi_vec, wci_vec, wei_vec, dwci_vec, Rei_vec, Phi_bar_psi_e_vec)
%%%% 计算补偿项
iiuav = 3;
Fi_S_3 = -cal_askew_mat( wi_vec(:,iiuav) ) * Ji(:,:,iiuav) * wi_vec(:,iiuav) ...
                + Ji(:,:,iiuav) * cal_askew_mat( wei_vec(:,iiuav) ) * ( Rei_vec(:,:,iiuav)' ) * wci_vec(:,iiuav) ...
                - Ji(:,:,iiuav) * ( Rei_vec(:,:,iiuav)' ) * dwci_vec(:,iiuav) ...
                + cS0 * Ji(:,:,iiuav) * Phi_bar_psi_e_vec(:,iiuav);

== matlab function sim_att_dist_obs_tie_2020/cal Fi_S agent 4 ==
  data: cS0 input; Ji input; wi_vec input; wci_vec input; wei_vec input; Fi_S_4 output; dwci_vec input; Rei_vec input; Phi_bar_psi_e_vec input
function Fi_S_4 = fcn(cS0, Ji, wi_vec, wci_vec, wei_vec, dwci_vec, Rei_vec, Phi_bar_psi_e_vec)
%%%% 计算补偿项
iiuav = 4;
Fi_S_4 = -cal_askew_mat( wi_vec(:,iiuav) ) * Ji(:,:,iiuav) * wi_vec(:,iiuav) ...
                + Ji(:,:,iiuav) * cal_askew_mat( wei_vec(:,iiuav) ) * ( Rei_vec(:,:,iiuav)' ) * wci_vec(:,iiuav) ...
                - Ji(:,:,iiuav) * ( Rei_vec(:,:,iiuav)' ) * dwci_vec(:,iiuav) ...
                + cS0 * Ji(:,:,iiuav) * Phi_bar_psi_e_vec(:,iiuav);

== matlab function sim_att_dist_obs_tie_2020/cal Fi_S agent 5 ==
  data: cS0 input; Ji input; wi_vec input; wci_vec input; wei_vec input; Fi_S_5 output; dwci_vec input; Rei_vec input; Phi_bar_psi_e_vec input
function Fi_S_5 = fcn(cS0, Ji, wi_vec, wci_vec, wei_vec, dwci_vec, Rei_vec, Phi_bar_psi_e_vec)
%%%% 计算补偿项
iiuav = 5;
Fi_S_5 = -cal_askew_mat( wi_vec(:,iiuav) ) * Ji(:,:,iiuav) * wi_vec(:,iiuav) ...
                + Ji(:,:,iiuav) * cal_askew_mat( wei_vec(:,iiuav) ) * ( Rei_vec(:,:,iiuav)' ) * wci_vec(:,iiuav) ...
                - Ji(:,:,iiuav) * ( Rei_vec(:,:,iiuav)' ) * dwci_vec(:,iiuav) ...
                + cS0 * Ji(:,:,iiuav) * Phi_bar_psi_e_vec(:,iiuav);

== matlab function sim_att_dist_obs_tie_2020/cal Phi_bar_psi_e agent 1 ==
  data: pp0 input; Phi_bar_psi_e_node_1 output; beta_Phi_1 input; beta_Phi_2 input; thr_p_plus_1 input; gamma0 input; eps_s_bar_div_pi input; wei_vec input; S_bar_vec input; V_Phi_Rei_div_pi_vec input; V_Phi_Rei_squ_p_min_1_vec input; V_Phi_Rei_squ_p_plus_1_vec input; V_Phi_Rei_squ_2p_vec input
function Phi_bar_psi_e_node_1 = fcn(pp0, beta_Phi_1, beta_Phi_2, thr_p_plus_1, gamma0, ...
                                                                    eps_s_bar_div_pi, wei_vec, S_bar_vec, V_Phi_Rei_div_pi_vec, ...
                                                                    V_Phi_Rei_squ_p_min_1_vec, V_Phi_Rei_squ_p_plus_1_vec, V_Phi_Rei_squ_2p_vec)
%%%% 计算姿态误差项
iiuav = 1;
Phi_bar_psi_e_node_1 = zeros(3,1);
for kk = 1:3
    if S_bar_vec(kk, iiuav) == 0
        Phi_bar_psi_e_node_1(kk, 1) = thr_p_plus_1 * ( pp0 + 1 ) * V_Phi_Rei_div_pi_vec(kk, iiuav) ...
                                                                * V_Phi_Rei_squ_p_min_1_vec(kk, iiuav) * wei_vec(kk, iiuav) ...
                                                                / ( 2 * tanh( ( gamma0 / 2 ) * V_Phi_Rei_div_pi_vec(kk, iiuav) ) ) ...
                                                                + ( thr_p_plus_1 * gamma0 / 4 ) * V_Phi_Rei_squ_p_plus_1_vec(kk, iiuav) ...
                                                                * ( ( sech( ( gamma0 / 2 ) * V_Phi_Rei_div_pi_vec(kk, iiuav) ) ...
                                                                / tanh( ( gamma0 / 2 ) * V_Phi_Rei_div_pi_vec(kk, iiuav) ) ) ^ 2 ) * wei_vec(kk, iiuav);
    else
        if abs( V_Phi_Rei_div_pi_vec ) > eps_s_bar_div_pi
            Phi_bar_psi_e_node_1(kk, 1) = thr_p_plus_1 * ( pp0 + 1 ) * V_Phi_Rei_div_pi_vec(kk, iiuav) ...
                                                                    * V_Phi_Rei_squ_p_min_1_vec(kk, iiuav) * wei_vec(kk, iiuav) ...
                                                                    / ( 2 * tanh( ( gamma0 / 2 ) * V_Phi_Rei_div_pi_vec(kk, iiuav) ) ) ...
                                                                    + ( thr_p_plus_1 * gamma0 / 4 ) * V_Phi_Rei_squ_p_plus_1_vec(kk, iiuav) ...
                                                                    * ( ( sech( ( gamma0 / 2 ) * V_Phi_Rei_div_pi_vec(kk, iiuav) ) ...
                                                                    / tanh( ( gamma0 / 2 ) * V_Phi_Rei_div_pi_vec(kk, iiuav) ) ) ^ 2 ) * wei_vec(kk, iiuav);
        else
            Phi_bar_psi_e_node_1(kk, 1) = 2 * beta_Phi_1 * ( ( abs( V_Phi_Rei_div_pi_vec(kk, iiuav) ) ) ^ 2 ) * wei_vec(kk, iiuav) ...
                                                                    + ( 2 * pp0 + 1 ) * beta_Phi_2 * V_Phi_Rei_squ_2p_vec(kk, iiuav) * wei_vec(kk, iiuav);
        end
    end
end

== matlab function sim_att_dist_obs_tie_2020/cal Phi_bar_psi_e agent 2 ==
  data: pp0 input; Phi_bar_psi_e_node_2 output; beta_Phi_1 input; beta_Phi_2 input; thr_p_plus_1 input; gamma0 input; eps_s_bar_div_pi input; wei_vec input; S_bar_vec input; V_Phi_Rei_div_pi_vec input; V_Phi_Rei_squ_p_min_1_vec input; V_Phi_Rei_squ_p_plus_1_vec input; V_Phi_Rei_squ_2p_vec input
function Phi_bar_psi_e_node_2 = fcn(pp0, beta_Phi_1, beta_Phi_2, thr_p_plus_1, gamma0, ...
                                                                    eps_s_bar_div_pi, wei_vec, S_bar_vec, V_Phi_Rei_div_pi_vec, ...
                                                                    V_Phi_Rei_squ_p_min_1_vec, V_Phi_Rei_squ_p_plus_1_vec, V_Phi_Rei_squ_2p_vec)
%%%% 计算姿态误差项
iiuav = 2;
Phi_bar_psi_e_node_2 = zeros(3,1);
for kk = 1:3
    if S_bar_vec(kk, iiuav) == 0
        Phi_bar_psi_e_node_2(kk, 1) = thr_p_plus_1 * ( pp0 + 1 ) * V_Phi_Rei_div_pi_vec(kk, iiuav) ...
                                                                * V_Phi_Rei_squ_p_min_1_vec(kk, iiuav) * wei_vec(kk, iiuav) ...
                                                                / ( 2 * tanh( ( gamma0 / 2 ) * V_Phi_Rei_div_pi_vec(kk, iiuav) ) ) ...
                                                                + ( thr_p_plus_1 * gamma0 / 4 ) * V_Phi_Rei_squ_p_plus_1_vec(kk, iiuav) ...
                                                                * ( ( sech( ( gamma0 / 2 ) * V_Phi_Rei_div_pi_vec(kk, iiuav) ) ...
                                                                / tanh( ( gamma0 / 2 ) * V_Phi_Rei_div_pi_vec(kk, iiuav) ) ) ^ 2 ) * wei_vec(kk, iiuav);
    else
        if abs( V_Phi_Rei_div_pi_vec ) > eps_s_bar_div_pi
            Phi_bar_psi_e_node_2(kk, 1) = thr_p_plus_1 * ( pp0 + 1 ) * V_Phi_Rei_div_pi_vec(kk, iiuav) ...
                                                                    * V_Phi_Rei_squ_p_min_1_vec(kk, iiuav) * wei_vec(kk, iiuav) ...
                                                                    / ( 2 * tanh( ( gamma0 / 2 ) * V_Phi_Rei_div_pi_vec(kk, iiuav) ) ) ...
                                                                    + ( thr_p_plus_1 * gamma0 / 4 ) * V_Phi_Rei_squ_p_plus_1_vec(kk, iiuav) ...
                                                                    * ( ( sech( ( gamma0 / 2 ) * V_Phi_Rei_div_pi_vec(kk, iiuav) ) ...
                                                                    / tanh( ( gamma0 / 2 ) * V_Phi_Rei_div_pi_vec(kk, iiuav) ) ) ^ 2 ) * wei_vec(kk, iiuav);
        else
            Phi_bar_psi_e_node_2(kk, 1) = 2 * beta_Phi_1 * ( ( abs( V_Phi_Rei_div_pi_vec(kk, iiuav) ) ) ^ 2 ) * wei_vec(kk, iiuav) ...
                                                                    + ( 2 * pp0 + 1 ) * beta_Phi_2 * V_Phi_Rei_squ_2p_vec(kk, iiuav) * wei_vec(kk, iiuav);
        end
    end
end

== matlab function sim_att_dist_obs_tie_2020/cal Phi_bar_psi_e agent 3 ==
  data: pp0 input; Phi_bar_psi_e_node_3 output; beta_Phi_1 input; beta_Phi_2 input; thr_p_plus_1 input; gamma0 input; eps_s_bar_div_pi input; wei_vec input; S_bar_vec input; V_Phi_Rei_div_pi_vec input; V_Phi_Rei_squ_p_min_1_vec input; V_Phi_Rei_squ_p_plus_1_vec input; V_Phi_Rei_squ_2p_vec input
function Phi_bar_psi_e_node_3 = fcn(pp0, beta_Phi_1, beta_Phi_2, thr_p_plus_1, gamma0, ...
                                                                    eps_s_bar_div_pi, wei_vec, S_bar_vec, V_Phi_Rei_div_pi_vec, ...
                                                                    V_Phi_Rei_squ_p_min_1_vec, V_Phi_Rei_squ_p_plus_1_vec, V_Phi_Rei_squ_2p_vec)
%%%% 计算姿态误差项
iiuav = 3;
Phi_bar_psi_e_node_3 = zeros(3,1);
for kk = 1:3
    if S_bar_vec(kk, iiuav) == 0
        Phi_bar_psi_e_node_3(kk, 1) = thr_p_plus_1 * ( pp0 + 1 ) * V_Phi_Rei_div_pi_vec(kk, iiuav) ...
                                                                * V_Phi_Rei_squ_p_min_1_vec(kk, iiuav) * wei_vec(kk, iiuav) ...
                                                                / ( 2 * tanh( ( gamma0 / 2 ) * V_Phi_Rei_div_pi_vec(kk, iiuav) ) ) ...
                                                                + ( thr_p_plus_1 * gamma0 / 4 ) * V_Phi_Rei_squ_p_plus_1_vec(kk, iiuav) ...
                                                                * ( ( sech( ( gamma0 / 2 ) * V_Phi_Rei_div_pi_vec(kk, iiuav) ) ...
                                                                / tanh( ( gamma0 / 2 ) * V_Phi_Rei_div_pi_vec(kk, iiuav) ) ) ^ 2 ) * wei_vec(kk, iiuav);
    else
        if abs( V_Phi_Rei_div_pi_vec ) > eps_s_bar_div_pi
            Phi_bar_psi_e_node_3(kk, 1) = thr_p_plus_1 * ( pp0 + 1 ) * V_Phi_Rei_div_pi_vec(kk, iiuav) ...
                                                                    * V_Phi_Rei_squ_p_min_1_vec(kk, iiuav) * wei_vec(kk, iiuav) ...
                                                                    / ( 2 * tanh( ( gamma0 / 2 ) * V_Phi_Rei_div_pi_vec(kk, iiuav) ) ) ...
                                                                    + ( thr_p_plus_1 * gamma0 / 4 ) * V_Phi_Rei_squ_p_plus_1_vec(kk, iiuav) ...
                                                                    * ( ( sech( ( gamma0 / 2 ) * V_Phi_Rei_div_pi_vec(kk, iiuav) ) ...
                                                                    / tanh( ( gamma0 / 2 ) * V_Phi_Rei_div_pi_vec(kk, iiuav) ) ) ^ 2 ) * wei_vec(kk, iiuav);
        else
            Phi_bar_psi_e_node_3(kk, 1) = 2 * beta_Phi_1 * ( ( abs( V_Phi_Rei_div_pi_vec(kk, iiuav) ) ) ^ 2 ) * wei_vec(kk, iiuav) ...
                                                                    + ( 2 * pp0 + 1 ) * beta_Phi_2 * V_Phi_Rei_squ_2p_vec(kk, iiuav) * wei_vec(kk, iiuav);
        end
    end
end

== matlab function sim_att_dist_obs_tie_2020/cal Phi_bar_psi_e agent 4 ==
  data: pp0 input; Phi_bar_psi_e_node_4 output; beta_Phi_1 input; beta_Phi_2 input; thr_p_plus_1 input; gamma0 input; eps_s_bar_div_pi input; wei_vec input; S_bar_vec input; V_Phi_Rei_div_pi_vec input; V_Phi_Rei_squ_p_min_1_vec input; V_Phi_Rei_squ_p_plus_1_vec input; V_Phi_Rei_squ_2p_vec input
function Phi_bar_psi_e_node_4 = fcn(pp0, beta_Phi_1, beta_Phi_2, thr_p_plus_1, gamma0, ...
                                                                    eps_s_bar_div_pi, wei_vec, S_bar_vec, V_Phi_Rei_div_pi_vec, ...
                                                                    V_Phi_Rei_squ_p_min_1_vec, V_Phi_Rei_squ_p_plus_1_vec, V_Phi_Rei_squ_2p_vec)
%%%% 计算姿态误差项
iiuav = 4;
Phi_bar_psi_e_node_4 = zeros(3,1);
for kk = 1:3
    if S_bar_vec(kk, iiuav) == 0
        Phi_bar_psi_e_node_4(kk, 1) = thr_p_plus_1 * ( pp0 + 1 ) * V_Phi_Rei_div_pi_vec(kk, iiuav) ...
                                                                * V_Phi_Rei_squ_p_min_1_vec(kk, iiuav) * wei_vec(kk, iiuav) ...
                                                                / ( 2 * tanh( ( gamma0 / 2 ) * V_Phi_Rei_div_pi_vec(kk, iiuav) ) ) ...
                                                                + ( thr_p_plus_1 * gamma0 / 4 ) * V_Phi_Rei_squ_p_plus_1_vec(kk, iiuav) ...
                                                                * ( ( sech( ( gamma0 / 2 ) * V_Phi_Rei_div_pi_vec(kk, iiuav) ) ...
                                                                / tanh( ( gamma0 / 2 ) * V_Phi_Rei_div_pi_vec(kk, iiuav) ) ) ^ 2 ) * wei_vec(kk, iiuav);
    else
        if abs( V_Phi_Rei_div_pi_vec ) > eps_s_bar_div_pi
            Phi_bar_psi_e_node_4(kk, 1) = thr_p_plus_1 * ( pp0 + 1 ) * V_Phi_Rei_div_pi_vec(kk, iiuav) ...
                                                                    * V_Phi_Rei_squ_p_min_1_vec(kk, iiuav) * wei_vec(kk, iiuav) ...
                                                                    / ( 2 * tanh( ( gamma0 / 2 ) * V_Phi_Rei_div_pi_vec(kk, iiuav) ) ) ...
                                                                    + ( thr_p_plus_1 * gamma0 / 4 ) * V_Phi_Rei_squ_p_plus_1_vec(kk, iiuav) ...
                                                                    * ( ( sech( ( gamma0 / 2 ) * V_Phi_Rei_div_pi_vec(kk, iiuav) ) ...
                                                                    / tanh( ( gamma0 / 2 ) * V_Phi_Rei_div_pi_vec(kk, iiuav) ) ) ^ 2 ) * wei_vec(kk, iiuav);
        else
            Phi_bar_psi_e_node_4(kk, 1) = 2 * beta_Phi_1 * ( ( abs( V_Phi_Rei_div_pi_vec(kk, iiuav) ) ) ^ 2 ) * wei_vec(kk, iiuav) ...
                                                                    + ( 2 * pp0 + 1 ) * beta_Phi_2 * V_Phi_Rei_squ_2p_vec(kk, iiuav) * wei_vec(kk, iiuav);
        end
    end
end
